simulink model "test_4"  (R2018a)
settings: Solver=ode4  StartTime=0.0  StopTime=10.0  FixedStep=1e-3  RelTol=1e-3
settings Model: Creator=wol4aravio  LastModifiedBy=wol4aravio

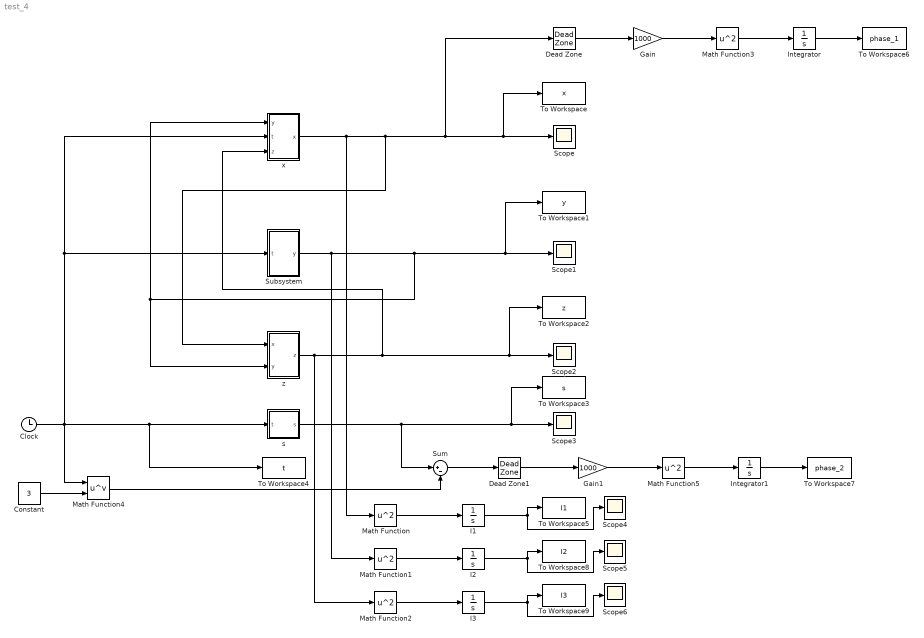
== system test_4 ==
  Clock : Clock
  Constant : Constant  Value=3
  Dead Zone : DeadZone  LowerValue=-inf  UpperValue=0.0  SaturateOnIntegerOverflow=on
  Dead Zone1 : DeadZone  LowerValue=-inf  UpperValue=0.0  SaturateOnIntegerOverflow=on
  Gain : Gain  Gain=1000
  Gain1 : Gain  Gain=1000
  I1 : Integrator  ContinuousStateAttributes='y'
  I2 : Integrator  ContinuousStateAttributes='y'
  I3 : Integrator  ContinuousStateAttributes='y'
  Integrator : Integrator
  Integrator1 : Integrator
  Math Function{,1..3,5} (5 alike) : Math  Operator=square  SaturateOnIntegerOverflow=on
  Math Function4 : Math  Operator=pow  SaturateOnIntegerOverflow=on
  Scope{,1..6} (7 alike) : Scope
  Subsystem : Subsystem
  Sum : Sum  Inputs=|+-
  To Workspace : ToWorkspace  VariableName=x  SaveFormat=Timeseries  SampleTime=-1
  To Workspace1 : ToWorkspace  VariableName=y  SaveFormat=Timeseries  SampleTime=-1
  To Workspace2 : ToWorkspace  VariableName=z  SaveFormat=Timeseries  SampleTime=-1
  To Workspace3 : ToWorkspace  VariableName=s  SaveFormat=Timeseries  SampleTime=-1
  To Workspace4 : ToWorkspace  VariableName=t  SaveFormat=Timeseries  SampleTime=-1
  To Workspace5 : ToWorkspace  VariableName=I1  SaveFormat=Timeseries  SampleTime=-1
  To Workspace6 : ToWorkspace  VariableName=phase_1  SaveFormat=Timeseries  SampleTime=-1
  To Workspace7 : ToWorkspace  VariableName=phase_2  SaveFormat=Timeseries  SampleTime=-1
  To Workspace8 : ToWorkspace  VariableName=I2  SaveFormat=Timeseries  SampleTime=-1
  To Workspace9 : ToWorkspace  VariableName=I3  SaveFormat=Timeseries  SampleTime=-1
  s : Subsystem
  x : Subsystem
  z : Subsystem
  wires:
  Clock/1 -> Math Function4/1, x/2(t), Subsystem/1(t), To Workspace4/1, s/1(t)
  Subsystem/1(y) -> Math Function1/1, To Workspace1/1, Scope1/1, x/1(y), z/2(y)
  z/1(z) -> Math Function2/1, To Workspace2/1, Scope2/1, x/3(z)
  x/1(x) -> Math Function/1, Dead Zone/1, To Workspace/1, Scope/1, z/1(x)
  s/1(s) -> Sum/1, To Workspace3/1, Scope3/1
  I1/1 -> Scope4/1, To Workspace5/1
  Dead Zone/1 -> Gain/1
  Gain/1 -> Math Function3/1
  Math Function3/1 -> Integrator/1
  Integrator/1 -> To Workspace6/1
  Constant/1 -> Math Function4/2
  Math Function4/1 -> Sum/2
  Integrator1/1 -> To Workspace7/1
  Math Function5/1 -> Integrator1/1
  Gain1/1 -> Math Function5/1
  Dead Zone1/1 -> Gain1/1
  Sum/1 -> Dead Zone1/1
  Math Function/1 -> I1/1
  I2/1 -> Scope5/1, To Workspace8/1
  Math Function1/1 -> I2/1
  I3/1 -> Scope6/1, To Workspace9/1
  Math Function2/1 -> I3/1

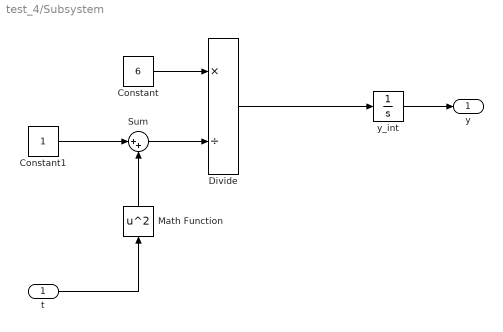
== system test_4/Subsystem ==
  t : Inport
  Constant : Constant  Value=6
  Constant1 : Constant
  Divide : Product  Inputs=*/
  Math Function : Math  Operator=square  SaturateOnIntegerOverflow=on
  Sum : Sum  Inputs=|++
  y_int : Integrator  ContinuousStateAttributes='y'
  y : Outport
  wires:
  Divide/1 -> y_int/1
  Math Function/1 -> Sum/2
  Sum/1 -> Divide/2
  t/1 -> Math Function/1
  Constant1/1 -> Sum/1
  y_int/1 -> y/1
  Constant/1 -> Divide/1

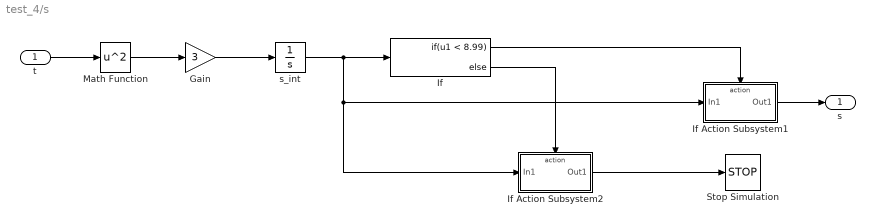
== system test_4/s ==
  t : Inport
  Gain : Gain  Gain=3
  If : If  IfExpression=u1 < 8.99
  If Action Subsystem1 : Subsystem  TreatAsAtomicUnit=on
  If Action Subsystem2 : Subsystem  TreatAsAtomicUnit=on
  Math Function : Math  Operator=square  SaturateOnIntegerOverflow=on
  Stop Simulation : Stop
  s_int : Integrator  ContinuousStateAttributes='s'
  s : Outport
  wires:
  s_int/1 -> If Action Subsystem2/1(In1), If Action Subsystem1/1(In1), If/1
  If/2 -> If Action Subsystem2/Action
  t/1 -> Math Function/1
  If/1 -> If Action Subsystem1/Action
  Math Function/1 -> Gain/1
  If Action Subsystem2/1(Out1) -> Stop Simulation/1
  If Action Subsystem1/1(Out1) -> s/1
  Gain/1 -> s_int/1

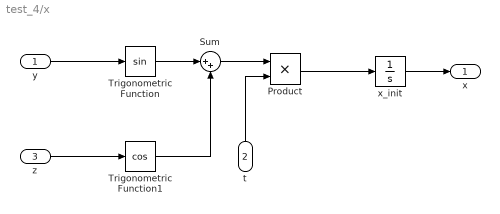
== system test_4/x ==
  y : Inport
  t : Inport  Port=2
  z : Inport  Port=3
  Product : Product
  Sum : Sum  Inputs=|++
  Trigonometric Function : Trigonometry
  Trigonometric Function1 : Trigonometry  Operator=cos
  x_init : Integrator  ContinuousStateAttributes='x'
  x : Outport
  wires:
  y/1 -> Trigonometric Function/1
  Trigonometric Function/1 -> Sum/1
  t/1 -> Product/2
  z/1 -> Trigonometric Function1/1
  Trigonometric Function1/1 -> Sum/2
  x_init/1 -> x/1
  Sum/1 -> Product/1
  Product/1 -> x_init/1

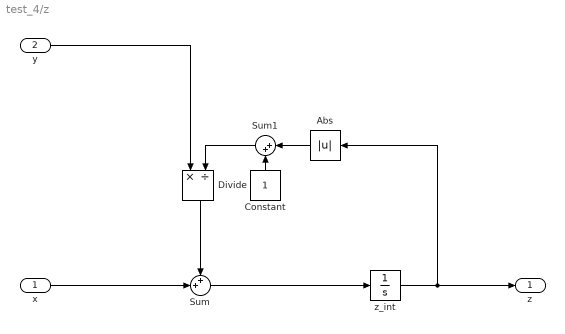
== system test_4/z ==
  x : Inport
  y : Inport  Port=2
  Abs : Abs
  Constant : Constant
  Divide : Product  Inputs=*/
  Sum : Sum  Inputs=++|
  Sum1 : Sum  Inputs=|++
  z_int : Integrator  ContinuousStateAttributes='z'
  z : Outport
  wires:
  y/1 -> Divide/1
  Sum/1 -> z_int/1
  x/1 -> Sum/2
  Abs/1 -> Sum1/1
  Constant/1 -> Sum1/2
  Divide/1 -> Sum/1
  Sum1/1 -> Divide/2
  z_int/1 -> z/1, Abs/1

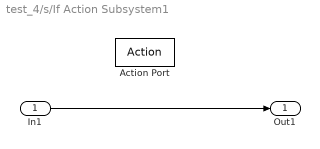
== system test_4/s/If Action Subsystem1 ==
  In1 : Inport
  Action Port : ActionPort  ActionType=then
  Out1 : Outport
  wires:
  In1/1 -> Out1/1

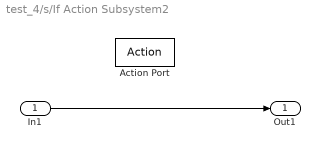
== system test_4/s/If Action Subsystem2 ==
  In1 : Inport
  Action Port : ActionPort  ActionType=else
  Out1 : Outport
  wires:
  In1/1 -> Out1/1
